simulink model "introductionTaskPlusPotentiometer_tIB"  (R2014b)
settings: Solver=FixedStepDiscrete  StartTime=0.0  StopTime=10.0  RelTol=1e-3
libraries: c2833xlib x10, c280xlib x2
settings Model: Creator=Michael  LastModifiedBy=Michael
settings DataIOCC: SaveOutput=off  SaveTime=off
settings OptimizationCC: OptimizeModelRefInitCode=on  LifeSpan=1
settings HardwareCC: ProdBitPerChar=16  ProdBitPerInt=16  ProdBitPerPointer=16  ProdLargestAtomicInteger=Integer  ProdIntDivRoundTo=Zero  ProdEndianess=LittleEndian  ProdWordSize=16  ProdHWDeviceType=Texas Instruments->C2000
settings RTWCC: SystemTargetFile=idelink_ert.tlc  GenerateMakefile=off  TemplateMakefile=none  Description=IDE Link ERT  ProcessScript=idelink_ert_make_rtw_hook  Toolchain=Texas Instruments Code Composer Studio v5 (C2000)
settings CodeAppCC: IgnoreCustomStorageClasses=off
settings TargetHardwareResources: Description=Target Hardware Resources Component

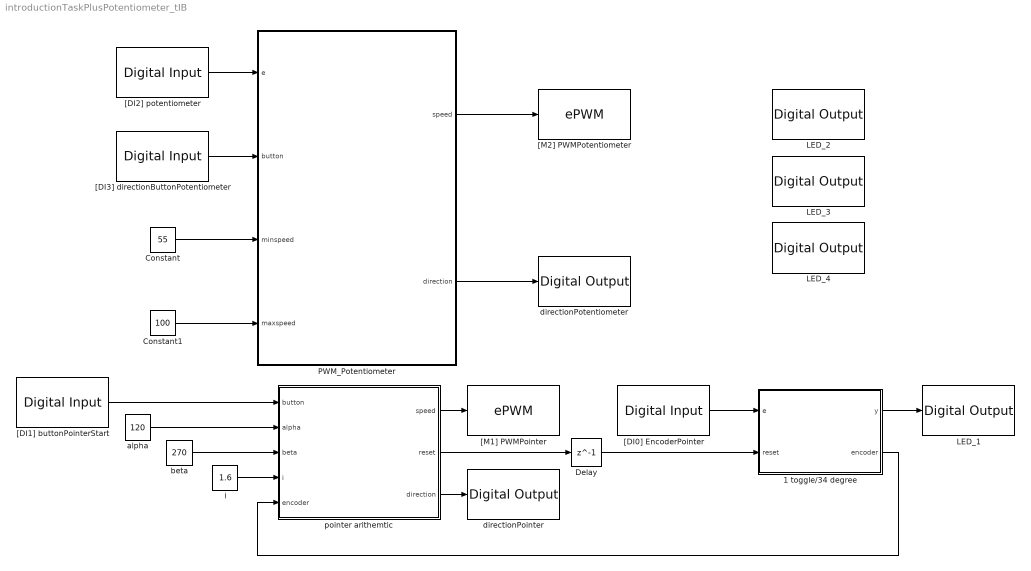
== system introductionTaskPlusPotentiometer_tIB ==
  1 toggle/34 degree : Stateflow chart  TreatAsAtomicUnit=on
  Constant : Constant  Value=55  OutMin=[0]  OutMax=[100]  OutDataTypeStr=uint16
  Constant1 : Constant  Value=100  OutMin=[0]  OutMax=[100]  OutDataTypeStr=uint16
  Delay : Delay  DelayLength=1  InitialCondition=0
  LED_1 : c2833xlib/Digital Output  GPIO_Number=GPIO56~GPIO63  GPIO_Bit0=off  GPIO_BIT0_Toggle=off  GPIO_Bit1=off  GPIO_BIT1_Toggle=off  GPIO_Bit2=on  GPIO_BIT2_Toggle=off  GPIO_Bit3=off  GPIO_BIT3_Toggle=off  GPIO_Bit4=off  GPIO_BIT4_Toggle=off  GPIO_Bit5=off  GPIO_BIT5_Toggle=off  GPIO_Bit6=off  GPIO_BIT6_Toggle=off  GPIO_Bit7=off  GPIO_BIT7_Toggle=off
  LED_2 : c2833xlib/Digital Output  GPIO_Number=GPIO56~GPIO63  GPIO_Bit0=off  GPIO_BIT0_Toggle=off  GPIO_Bit1=off  GPIO_BIT1_Toggle=off  GPIO_Bit2=off  GPIO_BIT2_Toggle=off  GPIO_Bit3=on  GPIO_BIT3_Toggle=on  GPIO_Bit4=off  GPIO_BIT4_Toggle=off  GPIO_Bit5=off  GPIO_BIT5_Toggle=off  GPIO_Bit6=off  GPIO_BIT6_Toggle=off  GPIO_Bit7=off  GPIO_BIT7_Toggle=off
  LED_3 : c2833xlib/Digital Output  GPIO_Number=GPIO56~GPIO63  GPIO_Bit0=off  GPIO_BIT0_Toggle=off  GPIO_Bit1=off  GPIO_BIT1_Toggle=off  GPIO_Bit2=off  GPIO_BIT2_Toggle=off  GPIO_Bit3=off  GPIO_BIT3_Toggle=off  GPIO_Bit4=on  GPIO_BIT4_Toggle=on  GPIO_Bit5=off  GPIO_BIT5_Toggle=off  GPIO_Bit6=off  GPIO_BIT6_Toggle=off  GPIO_Bit7=off  GPIO_BIT7_Toggle=off
  LED_4 : c2833xlib/Digital Output  GPIO_Number=GPIO56~GPIO63  GPIO_Bit0=off  GPIO_BIT0_Toggle=off  GPIO_Bit1=off  GPIO_BIT1_Toggle=off  GPIO_Bit2=off  GPIO_BIT2_Toggle=off  GPIO_Bit3=off  GPIO_BIT3_Toggle=off  GPIO_Bit4=off  GPIO_BIT4_Toggle=on  GPIO_Bit5=on  GPIO_BIT5_Toggle=on  GPIO_Bit6=off  GPIO_BIT6_Toggle=off  GPIO_Bit7=off  GPIO_BIT7_Toggle=off
  PWM_Potentiometer : Stateflow chart  TreatAsAtomicUnit=on
  "[DI0] EncoderPointer" : c2833xlib/Digital Input  GPIO_Number=GPIO24~GPIO31  GPIO_Bit0=on  GPIO_Bit1=off  GPIO_Bit2=off  GPIO_Bit3=off  GPIO_Bit4=off  GPIO_Bit5=off  GPIO_Bit6=off  GPIO_Bit7=off  sampleTime=0.001  dataType=auto  GPIO_Bit0_Qualification=Sync to SYSCLKOUT  GPIO_Bit1_Qualification=Sync to SYSCLKOUT  GPIO_Bit2_Qualification=Sync to SYSCLKOUT  GPIO_Bit3_Qualification=Sync to SYSCLKOUT  GPIO_Bit4_Qualification=Sync to SYSCLKOUT  GPIO_Bit5_Qualification=Sync to SYSCLKOUT  GPIO_Bit6_Qualification=Sync to SYSCLKOUT  GPIO_Bit7_Qualification=Sync to SYSCLKOUT  Qualification_Period=-1
  "[DI1] buttonPointerStart" : c2833xlib/Digital Input  GPIO_Number=GPIO24~GPIO31  GPIO_Bit0=off  GPIO_Bit1=on  GPIO_Bit2=off  GPIO_Bit3=off  GPIO_Bit4=off  GPIO_Bit5=off  GPIO_Bit6=off  GPIO_Bit7=off  sampleTime=0.001  dataType=auto  GPIO_Bit0_Qualification=Sync to SYSCLKOUT  GPIO_Bit1_Qualification=Sync to SYSCLKOUT  GPIO_Bit2_Qualification=Sync to SYSCLKOUT  GPIO_Bit3_Qualification=Sync to SYSCLKOUT  GPIO_Bit4_Qualification=Sync to SYSCLKOUT  GPIO_Bit5_Qualification=Sync to SYSCLKOUT  GPIO_Bit6_Qualification=Sync to SYSCLKOUT  GPIO_Bit7_Qualification=Sync to SYSCLKOUT  Qualification_Period=-1
  "[DI2] potentiometer" : c2833xlib/Digital Input  GPIO_Number=GPIO24~GPIO31  GPIO_Bit0=off  GPIO_Bit1=off  GPIO_Bit2=on  GPIO_Bit3=off  GPIO_Bit4=off  GPIO_Bit5=off  GPIO_Bit6=off  GPIO_Bit7=off  sampleTime=0.001  dataType=auto  GPIO_Bit0_Qualification=Sync to SYSCLKOUT  GPIO_Bit1_Qualification=Sync to SYSCLKOUT  GPIO_Bit2_Qualification=Sync to SYSCLKOUT  GPIO_Bit3_Qualification=Sync to SYSCLKOUT  GPIO_Bit4_Qualification=Sync to SYSCLKOUT  GPIO_Bit5_Qualification=Sync to SYSCLKOUT  GPIO_Bit6_Qualification=Sync to SYSCLKOUT  GPIO_Bit7_Qualification=Sync to SYSCLKOUT  Qualification_Period=-1
  "[DI3] directionButtonPotentiometer" : c2833xlib/Digital Input  GPIO_Number=GPIO24~GPIO31  GPIO_Bit0=off  GPIO_Bit1=off  GPIO_Bit2=off  GPIO_Bit3=on  GPIO_Bit4=off  GPIO_Bit5=off  GPIO_Bit6=off  GPIO_Bit7=off  sampleTime=0.001  dataType=auto  GPIO_Bit0_Qualification=Sync to SYSCLKOUT  GPIO_Bit1_Qualification=Sync to SYSCLKOUT  GPIO_Bit2_Qualification=Sync to SYSCLKOUT  GPIO_Bit3_Qualification=Sync to SYSCLKOUT  GPIO_Bit4_Qualification=Sync to SYSCLKOUT  GPIO_Bit5_Qualification=Sync to SYSCLKOUT  GPIO_Bit6_Qualification=Sync to SYSCLKOUT  GPIO_Bit7_Qualification=Sync to SYSCLKOUT  Qualification_Period=-1
  "[M1] PWMPointer" : c280xlib/ePWM  checkMode=off  useModule=ePWM2  periodUnits=Clock cycles  timerSource=Specify via dialog  timerPeriod_clk=64000  timerPeriod_sec=0.0001  tbshadow=Counter equals to zero  countingMode=Up  phaseActiveEnable=Disable  phaseDirection=Count down after sync  phaseActive=0  synchronizationEnable=off  synchronizationOption=Disable  clockPrescale=1  HSclockPrescale=1  ePWMxAStatus=off  CMPAUnits=Clock cycles  CMPASource=Specify via dialog  CMPAValue_per=50  CMPAValue_clk=32000  enCMPAshadow=Counter equals to zero  ePWMxAactionLogic1=Do nothing  ePWMxAactionLogic2=Clear  ePWMxAactionLogic3=Set  ePWMxAactionLogic4=Do nothing  ePWMxAactionLogic5=Do nothing  ePWMxAactionLogic6=Do nothing  ePWMxALoadMode=Load on counter equals to zero (CTR=Zero)  ePWMxACSFenable=off  ePWMxACSFvalue=Forcing disable  ePWMxASFreload=Zero  enHRPWM=off  HRPWM_LoadMode=Counter equals to zero (CTR=ZERO)  HRPWM_CTLMode=Phase control mode  HRPWM_EDGMode=Both edge  enSFO=on  ePWMxBStatus=on  CMPBUnits=Percentages  CMPBSource=Input port  CMPBValue_per=35  CMPBValue_clk=32000  enCMPBshadow=Counter equals to zero  ePWMxBactionLogic1=Do nothing  ePWMxBactionLogic2=Set  ePWMxBactionLogic3=Do nothing  ePWMxBactionLogic4=Do nothing  ePWMxBactionLogic5=Clear  ePWMxBactionLogic6=Do nothing  ePWMxBLoadMode=Load on counter equals to zero (CTR=Zero)  ePWMxBCSFenable=off  ePWMxBCSFvalue=Forcing disable  ePWMxBSFreload=Zero  enableDBePWMxA=off  enableDBePWMxB=off  DBpolarity=Active high (AH)  DBedgeDelay=Positive  DBSource_ePWMxA=ePWMxA  DBSource_ePWMxB=ePWMxA  DBperiodSource=Specify via dialog  REDperiod=0  FEDperiod=0  adcstartModuleA=off  adcrequestEventA=First event  adcstartEventA=Counter equals to zero (CTR=Zero)  adcstartModuleB=off  adcrequestEventB=First event  adcstartEventB=Counter equals to zero (CTR=Zero)  intEn=off  intPrd=First event  intSel=Counter equals to zero (CTR=Zero)  chopperEnable=off  chopperFrequency=1  chopperFirstwidth=1  chopperDuty=12.5%  tripZonesource=Specify via dialog  tzselOSHT1=off  tzselOSHT2=off  tzselOSHT3=off  tzselOSHT4=off  tzselOSHT5=off  tzselOSHT6=off  tzselCBC1=off  tzselCBC2=off  tzselCBC3=off  tzselCBC4=off  tzselCBC5=off  tzselCBC6=off  enTzOstIntr=off  enTzCbcIntr=off  ePWMxAforced=No action  ePWMxBforced=No action  timerPeriod=-1  ePWMxAValue=0  ePWMxBValue=0  tripZoneoption=One-shot trip (OSHT)
  "[M2] PWMPotentiometer" : c280xlib/ePWM  checkMode=off  useModule=ePWM1  periodUnits=Clock cycles  timerSource=Specify via dialog  timerPeriod_clk=64000  timerPeriod_sec=0.0001  tbshadow=Counter equals to zero  countingMode=Up  phaseActiveEnable=Disable  phaseDirection=Count down after sync  phaseActive=0  synchronizationEnable=off  synchronizationOption=Disable  clockPrescale=1  HSclockPrescale=1  ePWMxAStatus=off  CMPAUnits=Clock cycles  CMPASource=Specify via dialog  CMPAValue_per=50  CMPAValue_clk=32000  enCMPAshadow=Counter equals to zero  ePWMxAactionLogic1=Do nothing  ePWMxAactionLogic2=Clear  ePWMxAactionLogic3=Set  ePWMxAactionLogic4=Do nothing  ePWMxAactionLogic5=Do nothing  ePWMxAactionLogic6=Do nothing  ePWMxALoadMode=Load on counter equals to zero (CTR=Zero)  ePWMxACSFenable=off  ePWMxACSFvalue=Forcing disable  ePWMxASFreload=Zero  enHRPWM=off  HRPWM_LoadMode=Counter equals to zero (CTR=ZERO)  HRPWM_CTLMode=Phase control mode  HRPWM_EDGMode=Both edge  enSFO=on  ePWMxBStatus=on  CMPBUnits=Percentages  CMPBSource=Input port  CMPBValue_per=55  CMPBValue_clk=32000  enCMPBshadow=Counter equals to zero  ePWMxBactionLogic1=Do nothing  ePWMxBactionLogic2=Set  ePWMxBactionLogic3=Do nothing  ePWMxBactionLogic4=Do nothing  ePWMxBactionLogic5=Clear  ePWMxBactionLogic6=Do nothing  ePWMxBLoadMode=Load on counter equals to zero (CTR=Zero)  ePWMxBCSFenable=off  ePWMxBCSFvalue=Forcing disable  ePWMxBSFreload=Zero  enableDBePWMxA=off  enableDBePWMxB=off  DBpolarity=Active high (AH)  DBedgeDelay=Positive  DBSource_ePWMxA=ePWMxA  DBSource_ePWMxB=ePWMxA  DBperiodSource=Specify via dialog  REDperiod=0  FEDperiod=0  adcstartModuleA=off  adcrequestEventA=First event  adcstartEventA=Counter equals to zero (CTR=Zero)  adcstartModuleB=off  adcrequestEventB=First event  adcstartEventB=Counter equals to zero (CTR=Zero)  intEn=off  intPrd=First event  intSel=Counter equals to zero (CTR=Zero)  chopperEnable=off  chopperFrequency=1  chopperFirstwidth=1  chopperDuty=12.5%  tripZonesource=Specify via dialog  tzselOSHT1=off  tzselOSHT2=off  tzselOSHT3=off  tzselOSHT4=off  tzselOSHT5=off  tzselOSHT6=off  tzselCBC1=off  tzselCBC2=off  tzselCBC3=off  tzselCBC4=off  tzselCBC5=off  tzselCBC6=off  enTzOstIntr=off  enTzCbcIntr=off  ePWMxAforced=No action  ePWMxBforced=No action  timerPeriod=-1  ePWMxAValue=0  ePWMxBValue=0  tripZoneoption=One-shot trip (OSHT)
  alpha : Constant  Value=120  OutDataTypeStr=single
  beta : Constant  Value=270  OutDataTypeStr=single
  directionPointer : c2833xlib/Digital Output  GPIO_Number=GPIO16~GPIO23  GPIO_Bit0=off  GPIO_BIT0_Toggle=off  GPIO_Bit1=off  GPIO_BIT1_Toggle=off  GPIO_Bit2=off  GPIO_BIT2_Toggle=off  GPIO_Bit3=off  GPIO_BIT3_Toggle=off  GPIO_Bit4=off  GPIO_BIT4_Toggle=off  GPIO_Bit5=on  GPIO_BIT5_Toggle=off  GPIO_Bit6=off  GPIO_BIT6_Toggle=off  GPIO_Bit7=off  GPIO_BIT7_Toggle=off
  directionPotentiometer : c2833xlib/Digital Output  GPIO_Number=GPIO16~GPIO23  GPIO_Bit0=off  GPIO_BIT0_Toggle=off  GPIO_Bit1=off  GPIO_BIT1_Toggle=off  GPIO_Bit2=off  GPIO_BIT2_Toggle=off  GPIO_Bit3=off  GPIO_BIT3_Toggle=off  GPIO_Bit4=on  GPIO_BIT4_Toggle=off  GPIO_Bit5=off  GPIO_BIT5_Toggle=off  GPIO_Bit6=off  GPIO_BIT6_Toggle=off  GPIO_Bit7=off  GPIO_BIT7_Toggle=off
  i : Constant  Value=1.6  OutDataTypeStr=single
  pointer arithemtic : Stateflow chart  TreatAsAtomicUnit=on
  wires:
  alpha/1 -> pointer arithemtic/2(alpha)
  beta/1 -> pointer arithemtic/3(beta)
  i/1 -> pointer arithemtic/4(i)
  pointer arithemtic/1(speed) -> "[M1] PWMPointer"/1
  pointer arithemtic/2(reset) -> Delay/1
  "[DI0] EncoderPointer"/1 -> 1 toggle/34 degree/1(e)
  1 toggle/34 degree/1(y) -> LED_1/1
  1 toggle/34 degree/2(encoder) -> pointer arithemtic/5(encoder)
  Delay/1 -> 1 toggle/34 degree/2(reset)
  pointer arithemtic/3(direction) -> directionPointer/1
  "[DI1] buttonPointerStart"/1 -> pointer arithemtic/1(button)
  "[DI3] directionButtonPotentiometer"/1 -> PWM_Potentiometer/2(button)
  PWM_Potentiometer/2(direction) -> directionPotentiometer/1
  PWM_Potentiometer/1(speed) -> "[M2] PWMPotentiometer"/1
  "[DI2] potentiometer"/1 -> PWM_Potentiometer/1(e)
  Constant/1 -> PWM_Potentiometer/3(minspeed)
  Constant1/1 -> PWM_Potentiometer/4(maxspeed)

== stateflow chart introductionTaskPlusPotentiometer_tIB/1 toggle//34 degree ==
  state Drehung
    entry: y=~y;
    counter = int16(0);
  state X0
    entry: encoder= int16(0);
    counter = int16(0);
    y=false;
  state Start
    entry: encoder = encoder + 1;
    counter = counter + 1;
  state Ende
  Start -> Drehung [order 3] : [counter>=7]
  Drehung -> Start
  Start -> Ende [order 2] : [e>0]
  (default) -> X0
  X0 -> Start : [e>0]
  Ende -> Start : [e==0]
  Start -> X0 [order 1] : [reset==1]
  data: y output boolean; encoder output int16; e input; reset input; counter local int16

== stateflow chart introductionTaskPlusPotentiometer_tIB/PWM_Potentiometer ==
  state Speed_Controller [parallel]
    settings: executionOrder=2
    state Start
    state decelerate
      state start
      state reverse
        entry: direction = ~direction;
        reversed = true;
        accelerate_with_button = true;
      state decrease_speed
        entry: speed = speed - 1;
      state end
      (default) -> Speed_Controller.decelerate.start
      Speed_Controller.decelerate.start -> reverse [order 2] : [speed == minspeed]
      Speed_Controller.decelerate.start -> decrease_speed [order 1] : [speed > minspeed]
      decrease_speed -> Speed_Controller.decelerate.end
      reverse -> Speed_Controller.decelerate.end
    state accelerate
      state start
      state increase_speed
        entry: speed = speed + 1
      state end
      (default) -> Speed_Controller.accelerate.start
      Speed_Controller.accelerate.start -> Speed_Controller.accelerate.end [order 2] : [speed == maxspeed]
      Speed_Controller.accelerate.start -> increase_speed [order 1] : [speed < maxspeed]
      increase_speed -> Speed_Controller.accelerate.end
    (default) -> Start : {speed = uint16(minspeed);
        | direction = true;
        | reversed = false;
        | accelerate_with_button = false;}
    Start -> accelerate [order 1] : [[[e > 0] && [button == false]] || [[e>0] && [button == true] && [accelerate_with_button == true]]]
    Start -> decelerate [order 2] : [[e > 0] && [button == true] && [accelerate_with_button == false]]
    Speed_Controller.decelerate.end -> Start : [e == 0]
    Speed_Controller.accelerate.end -> Start : [e == 0]
  state Button_Direction_Detector [parallel]
    settings: executionOrder=1
    state steady
    state reset_after_reversion
      entry: accelerate_with_button = false;
      reversed = false;
    (default) -> steady
    reset_after_reversion -> steady
    steady -> reset_after_reversion : [[button == false] && [reversed == true]]
  data: e input; button input; speed output uint16; direction output boolean; reversed local boolean; accelerate_with_button local boolean; minspeed input uint16 =55; maxspeed input uint16 =100

== stateflow chart introductionTaskPlusPotentiometer_tIB/pointer arithemtic ==
  state start
    entry: speed = 0;
    direction = false;
    reset = true;
    alpha_reached =  alpha / 360 * i * 75;
    beta_reached =  beta / 360 * i * 75;
  state wait_and_prepare
    entry: reset = true;
    direction = [beta_reached < alpha_reached];
    beta_reached = abs( alpha_reached - beta_reached);
    exit: reset = false;
  state move_1
    entry: reset = false;
    speed = 55;
  state angle_alpha
    entry: speed = 0;
  state move_2
    entry: speed = 55;
  state wait_1
  move_1 -> angle_alpha : [encoder>=alpha_reached]
  angle_alpha -> wait_and_prepare : [beta_reached ~= alpha_reached]
  start -> wait_1 : after(200,msec)
  wait_1 -> move_1 : [button==true]
  (default) -> start
  wait_and_prepare -> move_2 : after(2000,msec)
  move_2 -> start : [encoder>=beta_reached]
  data: button input; alpha input; beta input; i input; speed output; encoder input; alpha_reached local single; beta_reached local single; reset output boolean; direction output boolean
